simulink model "SIL_beamNG"  (R2025b)
settings: Solver=FixedStepDiscrete  StartTime=0.0  StopTime=inf  FixedStep=0.01  RelTol=1e-3
libraries: simulink_extras x1
settings Model: NumberOfSteps=10  Creator=Gabriel  LastModifiedBy=mateu
settings SFSimCC: SimCustomInitializer=SS_App_Init();  SimUserIncludeDirs=..\..\include
settings SFSimCC: SimCustomHeaderCode=|
  | #include "ss_app.h"
  | 
  | #include "ss_input_proc.h"
  | 
  | #include "ss_operation.h"
  | 
  | #include "ss_types.h"
  | 
  | #include "ss_calib.h"
  | 
  | #include "ss_timer.h"
  | 
  | #include "ss_inhibit_safety_conditions.h"
  | 
  | #include "co2.h"
  | 
  | #include "ss_fuel.h"
  | 
  | #include "ss_control.h"
settings SFSimCC: SimUserSources=|
  | ..\..\src\ss_operation.c
  | 
  | ..\..\src\ss_input_proc.c
  | 
  | ..\..\src\ss_app.c
  | 
  | ..\..\src\timer.c
  | 
  | ..\..\src\ss_inhibit_safety_conditions.c
  | 
  | ..\..\src\co2.c
  | 
  | ..\..\src\ss_control.c
  | 
  | ..\..\src\ss_fuel.c

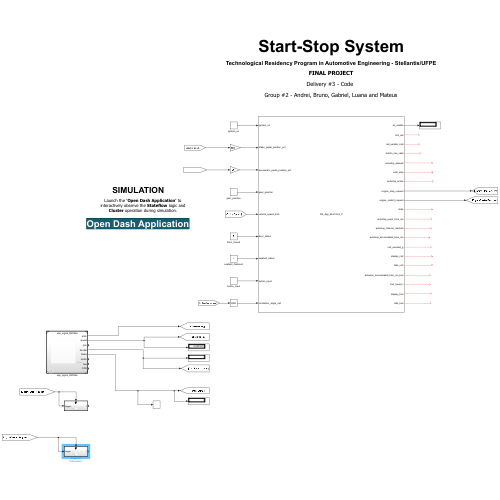
[thumbnail: Simulink's stored preview of the top-level diagram]
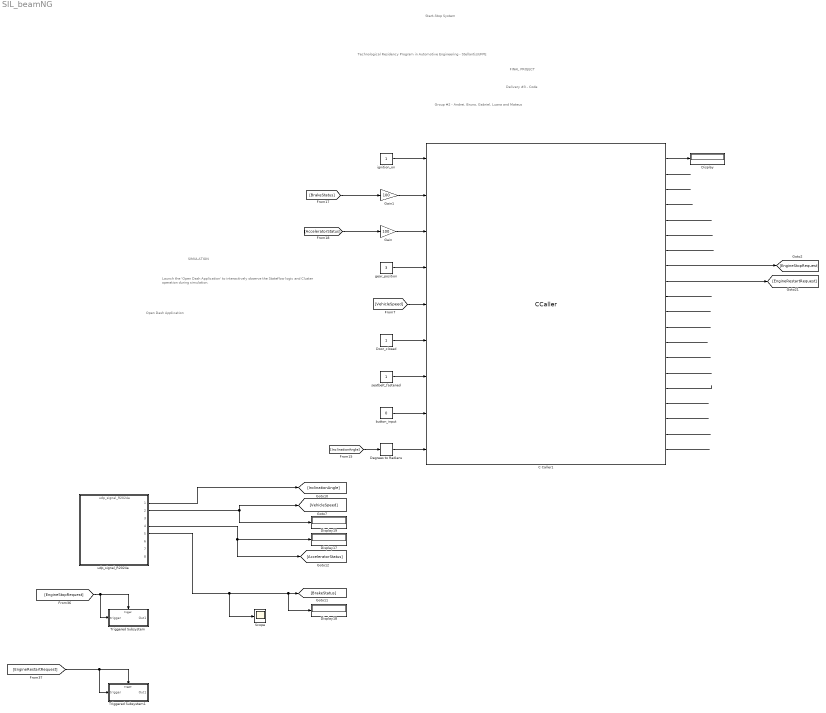
== system SIL_beamNG ==
  note: Open Dash Application
  note: Technological Residency Program in Automotive Engineering - Stellantis/UFPE
  note: Start-Stop System
  note: FINAL PROJECT
  note: Group #2 - Andrei, Bruno, Gabriel, Luana and Mateus
  note: Delivery #3 - Code
  note: SIMULATION
  note: Launch the 'Open Dash Application' to interactively observe the Stateflow logic and Cluster operation during simulation.
  C Caller1 : CCaller  FunctionName=SS_App_Run10ms_If  PortSpecificationStruct="%)30     .    ^#,   8    (     @         %    \"    !T    !     0         %  0 \"0    $    _    07)G3F%M90  4&]R=$YA;64 4V-O<&4     26YD97@     5'EP90      4VEZ90      27-';&]B86P   X   !     !@    @    $          4    (     0    L    !         !     +    :6=N:71I;VY?;VX       X   !     !@    @    $          4    (     0    L    !         !     +    :6=N:71I;VY?;VX       X    X    !@    @    $     ...(+17556 chars)"
  Degrees to Radians : simulink_extras/Transformations/Degrees to Radians
  Display{,17..19} (4 alike) : Display
  Door_closed : Constant  OutDataTypeStr=boolean
  Gain : Gain  Gain=100
  Gain1 : Gain  Gain=100
  Scope : Scope
      settings: TimeSpan=50  ActiveDisplayYMinimum=-1  ActiveDisplayYMaximum=1
  Triggered Subsystem : Subsystem  TreatAsAtomicUnit=on
  Triggered Subsystem1 : Subsystem  TreatAsAtomicUnit=on
  button_input : Constant  Value=0  OutDataTypeStr=boolean
  gear_position : Constant  Value=3  OutDataTypeStr=int32
  ignition_on : Constant  OutDataTypeStr=boolean
  seatbelt_fastened : Constant  OutDataTypeStr=boolean
  udp_signal_R2024a : ModelReference  ModelNameDialog=udp_signal_R2024a.slx  SimulationMode=Normal  ModelReferenceVersion=4.6
  wires:
  ignition_on/1 -> C Caller1/1
  C Caller1/1 -> Display/1
  C Caller1/8 -> [EngineStopRequest]
  C Caller1/9 -> [EngineRestartRequest]
  C Caller1/10 -> ?
  gear_position/1 -> C Caller1/4
  Door_closed/1 -> C Caller1/6
  seatbelt_fastened/1 -> C Caller1/7
  button_input/1 -> C Caller1/8
  udp_signal_R2024a/2 -> Display19/1, [VehicleSpeed]
  [VehicleSpeed] -> C Caller1/5
  [AcceleratorStatus] -> Gain/1
  [BrakeStatus] -> Gain1/1
  [EngineStopRequest] -> Triggered Subsystem/Trigger, Triggered Subsystem/1(trigger)
  udp_signal_R2024a/1 -> [InclinationAngle]
  C Caller1/5 -> ?
  C Caller1/7 -> ?
  Degrees to Radians/1 -> C Caller1/9
  C Caller1/6 -> ?
  [InclinationAngle] -> Degrees to Radians/1
  Gain/1 -> C Caller1/3
  Gain1/1 -> C Caller1/2
  C Caller1/11 -> ?
  C Caller1/12 -> ?
  C Caller1/13 -> ?
  C Caller1/14 -> ?
  C Caller1/15 -> ?
  C Caller1/16 -> ?
  C Caller1/17 -> ?
  C Caller1/18 -> ?
  C Caller1/19 -> ?
  C Caller1/20 -> ?
  C Caller1/2 -> ?
  C Caller1/3 -> ?
  C Caller1/4 -> ?
  udp_signal_R2024a/5 -> Scope/1, Display18/1, [BrakeStatus]
  udp_signal_R2024a/4 -> [AcceleratorStatus], Display17/1
  [EngineRestartRequest] -> Triggered Subsystem1/1(trigger), Triggered Subsystem1/Trigger

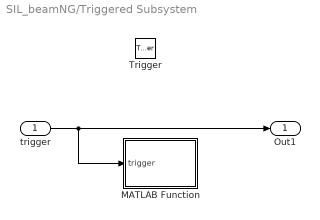
== system SIL_beamNG/Triggered Subsystem ==
  trigger : Inport
  Trigger : TriggerPort  VariantControl=(inherit)
  MATLAB Function : MATLAB Function  TreatAsAtomicUnit=on
  Out1 : Outport
  wires:
  trigger/1 -> MATLAB Function/1(trigger), Out1/1

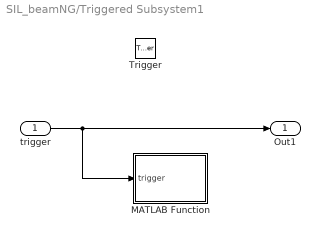
== system SIL_beamNG/Triggered Subsystem1 ==
  trigger : Inport
  Trigger : TriggerPort  VariantControl=(inherit)  InitialTriggerSignalState=zero
  MATLAB Function : MATLAB Function  TreatAsAtomicUnit=on
  Out1 : Outport
  wires:
  trigger/1 -> MATLAB Function/1(trigger), Out1/1

== matlab function SIL_beamNG/Triggered Subsystem1/MATLAB Function ==
  data: trigger input
function fcn(trigger)

%#codegen
coder.extrinsic('hold_v_key');

if trigger == 1
    hold_v_key();
end

== matlab function SIL_beamNG/Triggered Subsystem/MATLAB Function ==
  data: trigger input
function fcn(trigger)

%#codegen
coder.extrinsic('press_v_key');

if trigger == 1
    press_v_key();
    pause(0.25);
    press_v_key();
    pause(0.25);
    press_v_key();
    pause(0.25);
    press_v_key();
end
